simulink model "sampleModel1606_4_sub_sub"  (R2023a)
settings: Solver=VariableStepAuto  StartTime=0.0  StopTime=10.0  RelTol=1e-3
libraries: hdlsllib x6, simulink x3
settings Model: Creator=user1  LastModifiedBy=user1

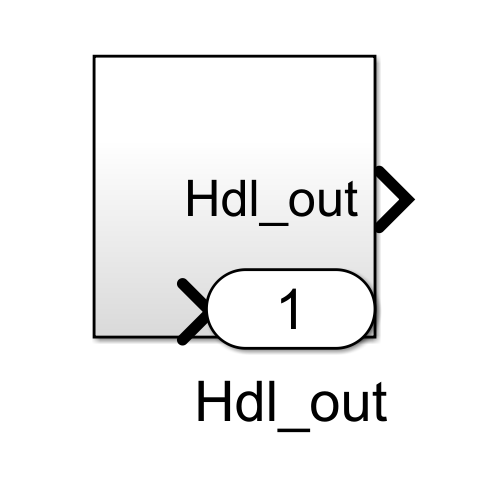
[thumbnail: Simulink's stored preview of the top-level diagram]
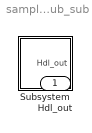
== system sampleModel1606_4_sub_sub ==
  Subsystem : Subsystem
  Hdl_out : Outport  OutDataTypeStr=uint8

== system sampleModel1606_4_sub_sub/Subsystem ==
  Subsystem : Subsystem
  Hdl_out : Outport  OutDataTypeStr=uint8

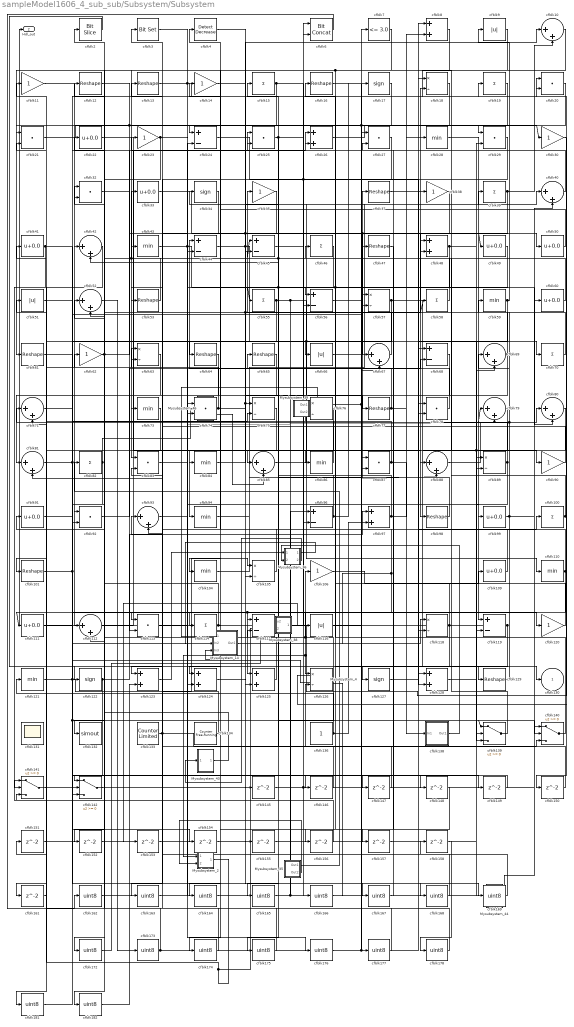
== system sampleModel1606_4_sub_sub/Subsystem/Subsystem ==
  Mysubsystem_14 : Subsystem  TreatAsAtomicUnit=on  RTWFcnName=Mysubsystem_14
      settings: RTWFcnNameOpts=User specified  RTWFileNameOpts=Use function name
  Mysubsystem_2 : Subsystem  TreatAsAtomicUnit=on  RTWFcnName=Mysubsystem_2
      settings: RTWFcnNameOpts=User specified  RTWFileNameOpts=Use function name
  Mysubsystem_35 : Subsystem  TreatAsAtomicUnit=on  RTWFcnName=Mysubsystem_35
      settings: RTWFcnNameOpts=User specified  RTWFileNameOpts=Use function name
  Mysubsystem_36 : Subsystem  TreatAsAtomicUnit=on  RTWFcnName=Mysubsystem_36
      settings: RTWFcnNameOpts=User specified  RTWFileNameOpts=Use function name
  Mysubsystem_38 : Subsystem  TreatAsAtomicUnit=on  RTWFcnName=Mysubsystem_38
      settings: RTWFcnNameOpts=User specified  RTWFileNameOpts=Use function name
  Mysubsystem_39 : Subsystem  TreatAsAtomicUnit=on  RTWFcnName=Mysubsystem_39
      settings: RTWFcnNameOpts=User specified  RTWFileNameOpts=Use function name
  Mysubsystem_4 : Subsystem  TreatAsAtomicUnit=on  RTWFcnName=Mysubsystem_4
      settings: RTWFcnNameOpts=User specified  RTWFileNameOpts=Use function name
  Mysubsystem_43 : Subsystem  TreatAsAtomicUnit=on  RTWFcnName=Mysubsystem_43
      settings: RTWFcnNameOpts=User specified  RTWFileNameOpts=Use function name
  Mysubsystem_44 : Subsystem  TreatAsAtomicUnit=on  RTWFcnName=Mysubsystem_44
      settings: RTWFcnNameOpts=User specified  RTWFileNameOpts=Use function name
  Mysubsystem_46 : Subsystem  TreatAsAtomicUnit=on  RTWFcnName=Mysubsystem_46
      settings: RTWFcnNameOpts=User specified  RTWFileNameOpts=Use function name
  cfblk{10,40,42,52,67,69,71,79..81,85,88,93,112} (14 alike) : Sum  Inputs=|++  OutDataTypeStr=uint8
  cfblk{15,19,39,46,55,58,70,82,100,114} (10 alike) : Sum  Inputs=+  OutDataTypeStr=uint8
  cfblk{12..13,16,37,47,53,61,64..65,77,98,101,129} (13 alike) : Reshape
  cfblk{28,43,59,73,84,86,94,104,110,121} (10 alike) : MinMax  OutDataTypeStr=uint8
  cfblk{18,57,63,75..76,89,105,118,126} (9 alike) : Product  Inputs=*/  OutDataTypeStr=uint8  RndMeth=Zero  SaturateOnIntegerOverflow=on
  cfblk{11,14,23,30,35,38,62,90,106,120} (10 alike) : Gain  OutDataTypeStr=uint8
  cfblk{22,33,41,49..50,60,91,99,109,111} (10 alike) : Bias  Bias=0.0  SaturateOnIntegerOverflow=off
  cfblk{20..21,25,27,29,32,74,78,83,87,92,113} (12 alike) : DotProduct  OutDataTypeStr=uint8
  cfblk{24,44..45,56,68,96,115,119} (8 alike) : Sum  Inputs=+-  OutDataTypeStr=uint8
  cfblk{9,51,66,116} (4 alike) : Abs  OutDataTypeStr=uint8  SaturateOnIntegerOverflow=off
  cfblk{17,34,122,127} (4 alike) : Signum
  cfblk{8,26,48,97,123..125,128} (8 alike) : Sum  OutDataTypeStr=uint8
  cfblk131 : Scope
      settings: Floating=on
  cfblk132 : ToWorkspace  VariableName=simout  SaveFormat=Timeseries  SampleTime=-1
  cfblk133 : hdlsllib/Sources/Counter Limited  uplimit=7  tsamp=-1
  cfblk134 : hdlsllib/Sources/Counter Free-Running  NumBits=16  tsamp=-1
  cfblk136 : Constant  OutDataTypeStr=uint8  SampleTime=-1
  cfblk138 : Subsystem
      settings: LibrarySourceBlock=|
      | hdlsllib/Ports &
      | Subsystems/Subsystem
  cfblk{139..142} (4 alike) : Switch  OutDataTypeStr=uint8  SaturateOnIntegerOverflow=off  InputSameDT=off
  cfblk{145..158,161} (15 alike) : Delay  SampleTime=1
  cfblk{162..169,172..178,181..182} (17 alike) : DataTypeConversion  OutDataTypeStr=uint8  SaturateOnIntegerOverflow=off  RndMeth=Floor
  cfblk2 : hdlsllib/Logic and Bit Operations/Bit Slice  lidx=7  ridx=0
  cfblk3 : simulink/Logic and Bit Operations/Bit Set  iBit=0
      settings: LibrarySourceBlock=|
      | hdlsllib/Logic and Bit
      | Operations/Bit Set
  cfblk4 : simulink/Logic and Bit Operations/Detect Decrease  vinit=0.0  OutDataTypeStr=uint8
      settings: LibrarySourceBlock=|
      | hdlsllib/Logic and Bit
      | Operations/Detect
      | Decrease
  cfblk6 : hdlsllib/Logic and Bit Operations/Bit Concat  numInputs=2
  cfblk7 : hdlsllib/Logic and Bit Operations/Compare To Constant  relop=<=  const=3.0  OutDataTypeStr=uint8
  cfblk130 : Outport  OutDataTypeStr=uint8  VectorParamsAs1DForOutWhenUnconnected=off
  Hdl_out : Outport  Port=2  OutDataTypeStr=uint8
  wires:
  Mysubsystem_46/1(Out1) -> cfblk85/2
  Mysubsystem_44/1(Out1) -> cfblk140/1
  Mysubsystem_4/1(Out1) -> Mysubsystem_44/1(In1)
  Mysubsystem_43/1(Out1) -> cfblk182/1
  Mysubsystem_36/2(Out2) -> Mysubsystem_43/1(In1)
  Mysubsystem_39/2(Out2) -> Mysubsystem_14/1(In1)
  Mysubsystem_39/1(Out1) -> cfblk19/1, cfblk88/2
  Mysubsystem_38/1(Out1) -> cfblk153/1
  cfblk172/1 -> Mysubsystem_38/1(u2)
  Mysubsystem_36/1(Out1) -> Mysubsystem_14/2(In2)
  cfblk138/1(Out1) -> Mysubsystem_36/2(In2)
  cfblk123/1 -> Mysubsystem_36/1(In1)
  Mysubsystem_35/2(Out2) -> Mysubsystem_2/2(In2)
  Mysubsystem_35/1(Out1) -> cfblk82/1
  Mysubsystem_14/1(Out1) -> cfblk81/2, Mysubsystem_2/1(In1), cfblk126/1
  cfblk181/1 -> Mysubsystem_4/2(In2)
  Mysubsystem_2/1(Out1) -> Mysubsystem_38/2(In2), cfblk141/3
  cfblk182/1 -> cfblk123/2
  cfblk73/1 -> cfblk181/1
  cfblk178/1 -> cfblk93/2
  cfblk158/1 -> cfblk178/1
  cfblk177/1 -> cfblk93/1
  cfblk16/1 -> cfblk177/1
  cfblk176/1 -> cfblk87/1, cfblk78/2
  cfblk175/1 -> cfblk52/2
  cfblk174/1 -> cfblk52/1
  cfblk35/1 -> cfblk174/1
  cfblk173/1 -> cfblk151/1, cfblk18/1
  cfblk169/1 -> cfblk158/1
  cfblk3/1 -> cfblk169/1
  cfblk168/1 -> cfblk3/1
  cfblk71/1 -> cfblk168/1
  cfblk167/1 -> cfblk27/2
  cfblk166/1 -> cfblk27/1
  cfblk165/1 -> cfblk69/2, cfblk96/1
  cfblk164/1 -> cfblk6/2
  cfblk148/1 -> cfblk164/1
  cfblk163/1 -> cfblk6/1
  cfblk68/1 -> cfblk163/1
  cfblk162/1 -> cfblk74/1
  cfblk6/1 -> cfblk162/1
  cfblk161/1 -> cfblk21/2
  cfblk157/1 -> cfblk128/1
  cfblk119/1 -> cfblk157/1, Hdl_out/1
  cfblk156/1 -> cfblk141/1
  cfblk155/1 -> cfblk78/1
  cfblk14/1 -> cfblk155/1
  cfblk154/1 -> cfblk89/1
  cfblk153/1 -> cfblk24/2
  cfblk152/1 -> cfblk68/1
  cfblk75/1 -> cfblk152/1
  cfblk151/1 -> cfblk74/2
  cfblk150/1 -> cfblk83/2
  cfblk30/1 -> cfblk150/1
  cfblk149/1 -> cfblk142/1
  cfblk61/1 -> cfblk149/1
  cfblk113/1 -> cfblk148/1
  cfblk147/1 -> cfblk115/2
  cfblk47/1 -> cfblk147/1
  cfblk146/1 -> cfblk126/2
  cfblk145/1 -> cfblk40/2
  cfblk124/1 -> cfblk145/1
  cfblk12/1 -> cfblk30/1, cfblk66/1
  cfblk64/1 -> cfblk92/1
  cfblk129/1 -> cfblk59/1, cfblk79/1
  cfblk116/1 -> cfblk57/1
  cfblk10/1 -> cfblk56/1, cfblk172/1
  cfblk34/1 -> cfblk53/1
  cfblk90/1 -> cfblk43/1
  cfblk141/1 -> cfblk118/1
  cfblk46/1 -> cfblk125/2
  cfblk139/1 -> cfblk48/1
  cfblk62/1 -> cfblk26/2, cfblk32/2
  cfblk53/1 -> cfblk12/1
  cfblk45/1 -> cfblk49/1, cfblk47/1
  cfblk82/1 -> Mysubsystem_46/1(In1), cfblk92/2
  cfblk133/1 -> cfblk63/2, cfblk140/3
  cfblk98/1 -> cfblk23/1
  cfblk128/1 -> cfblk140/2
  cfblk122/1 -> cfblk142/3, cfblk97/1
  cfblk69/1 -> cfblk32/1, cfblk71/2
  cfblk32/1 -> cfblk44/2
  cfblk109/1 -> cfblk63/1
  cfblk51/1 -> cfblk70/1
  cfblk4/1 -> cfblk75/1, cfblk167/1
  cfblk20/1 -> cfblk64/1
  cfblk101/1 -> cfblk130/1, cfblk75/2
  cfblk134/1 -> cfblk13/1
  cfblk83/1 -> cfblk96/2
  cfblk25/1 -> cfblk115/1, cfblk55/1, cfblk99/1
  cfblk74/1 -> cfblk51/1, cfblk77/1
  cfblk19/1 -> cfblk113/2, cfblk87/2
  cfblk48/1 -> cfblk124/2, cfblk50/1
  cfblk43/1 -> cfblk80/2, cfblk127/1
  cfblk96/1 -> cfblk34/1, cfblk45/1, cfblk17/1
  cfblk41/1 -> cfblk142/2, cfblk141/2
  cfblk97/1 -> cfblk42/2, cfblk28/1
  cfblk60/1 -> cfblk33/1, cfblk2/1
  cfblk50/1 -> cfblk14/1
  cfblk44/1 -> cfblk89/2, cfblk10/1
  cfblk110/1 -> cfblk125/1, cfblk111/1, cfblk71/1
  cfblk79/1 -> cfblk119/2, cfblk132/1
  cfblk66/1 -> cfblk67/2
  cfblk142/1 -> cfblk29/2, cfblk56/2
  cfblk106/1 -> cfblk109/1
  cfblk93/1 -> cfblk176/1
  cfblk49/1 -> cfblk124/1, cfblk146/1
  cfblk87/1 -> cfblk62/1, cfblk138/1(In1)
  cfblk29/1 -> cfblk113/1
  cfblk17/1 -> cfblk84/1
  cfblk15/1 -> cfblk21/1, cfblk88/1
  cfblk26/1 -> cfblk29/1
  cfblk33/1 -> cfblk67/1
  cfblk42/1 -> cfblk101/1
  cfblk111/1 -> cfblk20/2
  cfblk11/1 -> cfblk42/1
  cfblk40/1 -> cfblk25/1
  cfblk70/1 -> cfblk38/1
  cfblk92/1 -> cfblk68/2
  cfblk99/1 -> cfblk60/1, cfblk69/1
  cfblk114/1 -> Mysubsystem_14/3(In3), cfblk22/1
  cfblk125/1 -> cfblk91/1
  cfblk8/1 -> cfblk83/1
  cfblk38/1 -> cfblk123/1, cfblk45/2
  cfblk59/1 -> cfblk9/1, cfblk118/2
  cfblk127/1 -> cfblk100/1
  cfblk86/1 -> cfblk11/1
  cfblk84/1 -> cfblk39/1, cfblk58/1
  cfblk118/1 -> cfblk76/2, cfblk156/1
  cfblk22/1 -> cfblk85/1
  cfblk9/1 -> cfblk104/1
  cfblk65/1 -> cfblk114/1
  cfblk58/1 -> cfblk46/1
  cfblk81/1 -> cfblk120/1, cfblk57/2
  cfblk126/1 -> cfblk15/1, cfblk106/1, cfblk175/1
  cfblk120/1 -> cfblk76/1
  cfblk94/1 -> cfblk8/1
  cfblk21/1 -> cfblk24/1
  cfblk23/1 -> cfblk112/2, cfblk86/1
  cfblk77/1 -> cfblk44/1, cfblk8/2
  cfblk24/1 -> cfblk128/2, cfblk116/1
  cfblk140/1 -> cfblk16/1
  cfblk105/1 -> cfblk4/1
  cfblk91/1 -> cfblk139/1, cfblk154/1
  cfblk67/1 -> cfblk35/1
  cfblk115/1 -> cfblk20/1
  cfblk56/1 -> cfblk7/1
  cfblk39/1 -> cfblk98/1, cfblk10/2
  cfblk112/1 -> cfblk26/1
  cfblk85/1 -> cfblk40/1
  cfblk2/1 -> cfblk122/1
  cfblk89/1 -> cfblk41/1, cfblk139/3
  cfblk63/1 -> cfblk81/1
  cfblk57/1 -> cfblk90/1, cfblk161/1
  cfblk100/1 -> Mysubsystem_4/1(In1), cfblk48/2
  cfblk27/1 -> cfblk165/1
  cfblk136/1 -> cfblk121/1, cfblk97/2
  cfblk80/1 -> cfblk105/2
  cfblk78/1 -> cfblk65/1
  cfblk28/1 -> cfblk119/1
  cfblk55/1 -> cfblk110/1, cfblk139/2, cfblk166/1, cfblk73/1
  cfblk37/1 -> cfblk18/2
  cfblk52/1 -> cfblk173/1
  cfblk121/1 -> cfblk105/1, cfblk25/2
  cfblk104/1 -> cfblk37/1
  cfblk13/1 -> cfblk129/1, cfblk79/2
  cfblk88/1 -> cfblk80/1
  cfblk76/1 -> cfblk94/1
  cfblk7/1 -> cfblk61/1
  cfblk18/1 -> cfblk112/1

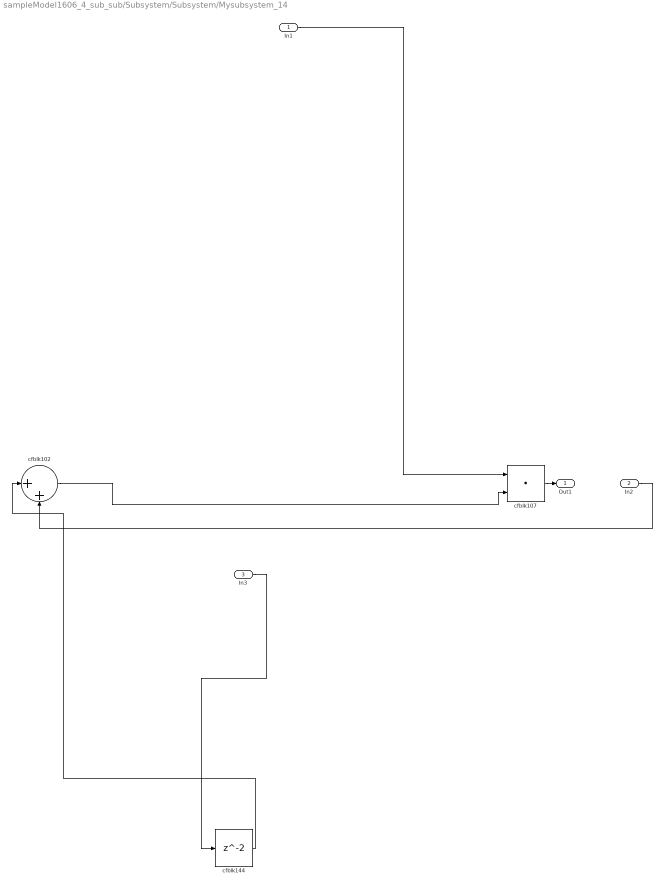
== system sampleModel1606_4_sub_sub/Subsystem/Subsystem/Mysubsystem_14 ==
  In1 : Inport
  In2 : Inport  Port=2
  In3 : Inport  Port=3
  cfblk102 : Sum  Inputs=|++
  cfblk107 : DotProduct  OutDataTypeStr=Inherit: Inherit via internal rule
  cfblk144 : Delay  SampleTime=1
  Out1 : Outport
  wires:
  cfblk102/1 -> cfblk107/2
  In2/1 -> cfblk102/2
  cfblk144/1 -> cfblk102/1
  In1/1 -> cfblk107/1
  cfblk107/1 -> Out1/1
  In3/1 -> cfblk144/1

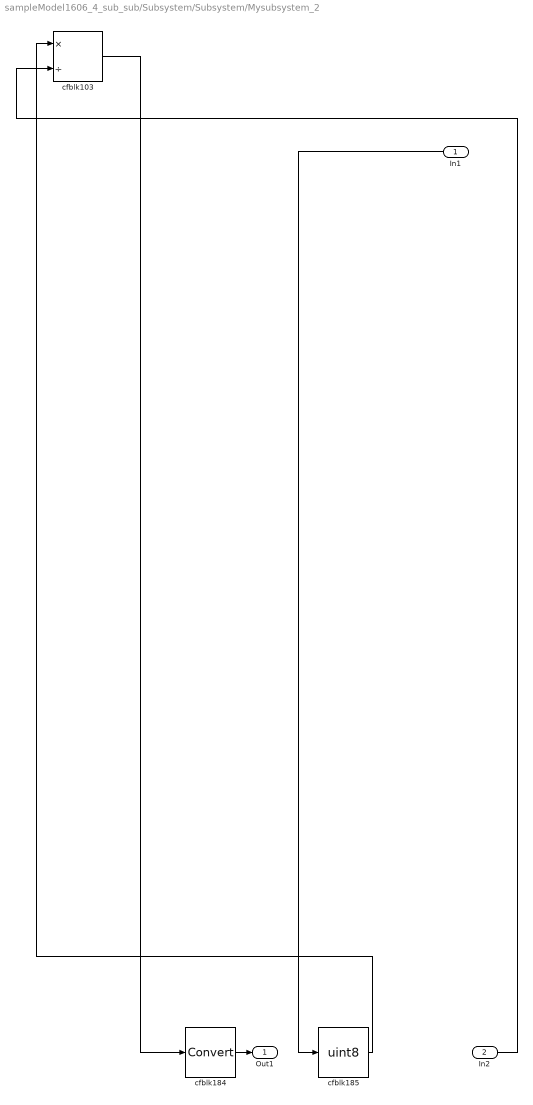
== system sampleModel1606_4_sub_sub/Subsystem/Subsystem/Mysubsystem_2 ==
  In1 : Inport
  In2 : Inport  Port=2
  cfblk103 : Product  Inputs=*/  RndMeth=Zero  SaturateOnIntegerOverflow=on
  cfblk184 : DataTypeConversion  SaturateOnIntegerOverflow=off  RndMeth=Floor
  cfblk185 : DataTypeConversion  OutDataTypeStr=uint8  SaturateOnIntegerOverflow=off  RndMeth=Floor
  Out1 : Outport
  wires:
  cfblk103/1 -> cfblk184/1
  cfblk185/1 -> cfblk103/1
  In2/1 -> cfblk103/2
  cfblk184/1 -> Out1/1
  In1/1 -> cfblk185/1

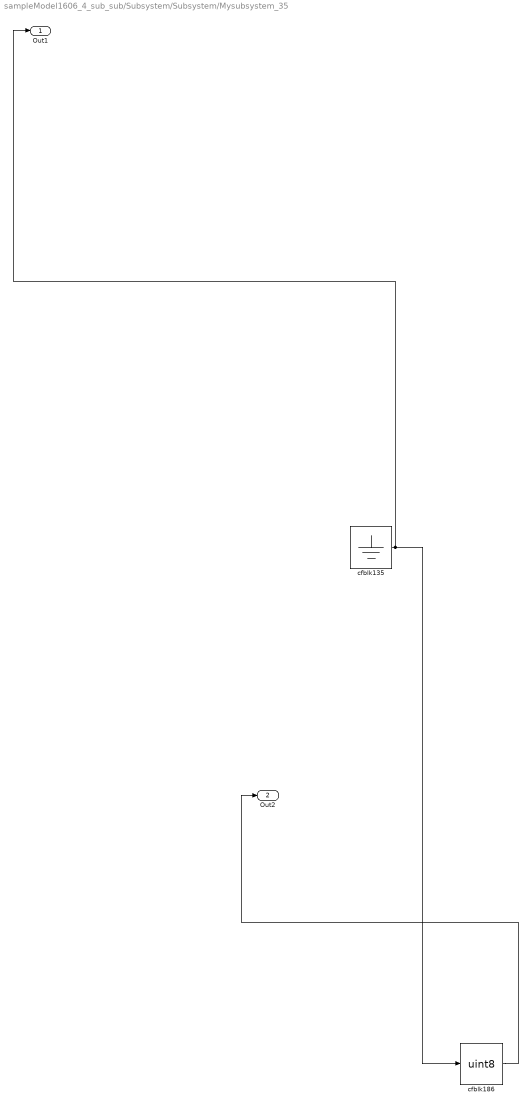
== system sampleModel1606_4_sub_sub/Subsystem/Subsystem/Mysubsystem_35 ==
  cfblk135 : Ground
  cfblk186 : DataTypeConversion  OutDataTypeStr=uint8  SaturateOnIntegerOverflow=off  RndMeth=Floor
  Out1 : Outport
  Out2 : Outport  Port=2
  wires:
  cfblk135/1 -> Out1/1, cfblk186/1
  cfblk186/1 -> Out2/1

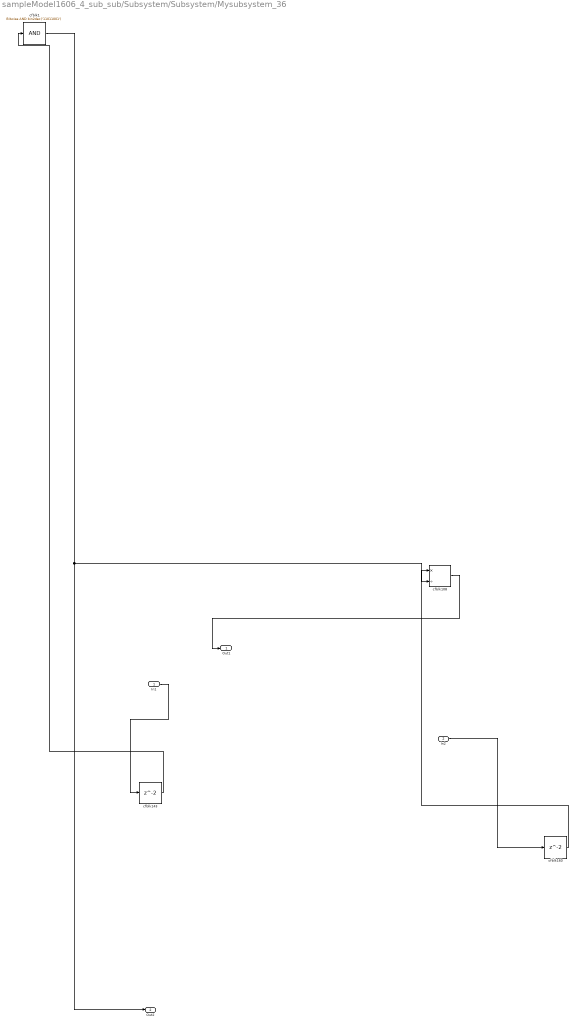
== system sampleModel1606_4_sub_sub/Subsystem/Subsystem/Mysubsystem_36 ==
  In1 : Inport
  In2 : Inport  Port=2
  cfblk1 : simulink/Logic and Bit Operations/Bitwise Operator  logicop=AND  UseBitMask=on  BitMask=bin2dec('11011001')  BitMaskRealWorld=Stored Integer
      settings: LibrarySourceBlock=|
      | hdlsllib/Logic and Bit
      | Operations/Bitwise
      | Operator
  cfblk108 : Product  Inputs=*/  RndMeth=Zero  SaturateOnIntegerOverflow=on
  cfblk143 : Delay  SampleTime=1
  cfblk160 : Delay  SampleTime=1
  Out1 : Outport
  Out2 : Outport  Port=2
  wires:
  cfblk1/1 -> Out2/1, cfblk108/2
  cfblk143/1 -> cfblk1/1
  cfblk160/1 -> cfblk108/1
  cfblk108/1 -> Out1/1
  In2/1 -> cfblk160/1
  In1/1 -> cfblk143/1

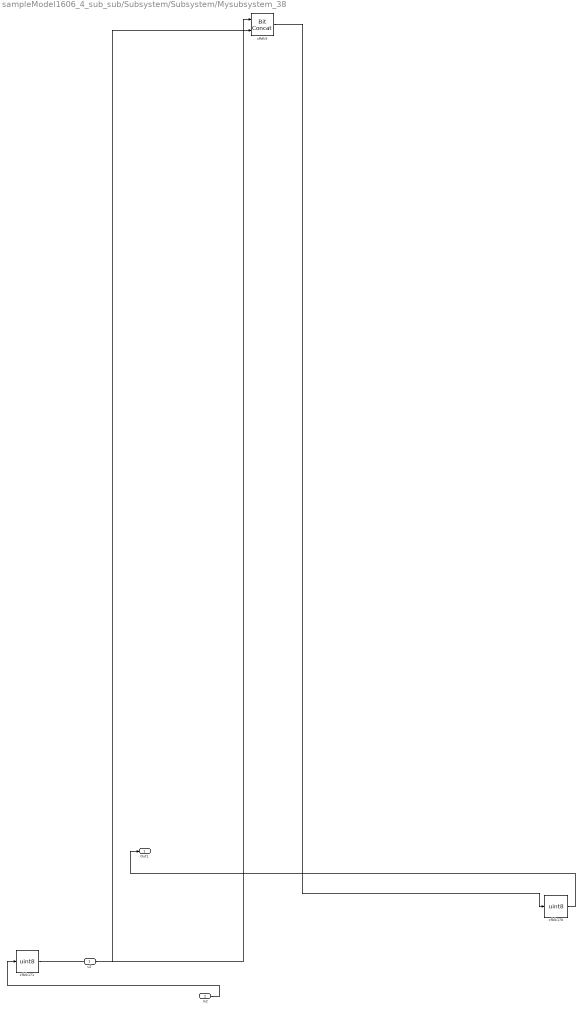
== system sampleModel1606_4_sub_sub/Subsystem/Subsystem/Mysubsystem_38 ==
  u2 : Inport
  In2 : Inport  Port=2
  cfblk170 : DataTypeConversion  OutDataTypeStr=uint8  SaturateOnIntegerOverflow=off  RndMeth=Floor
  cfblk171 : DataTypeConversion  OutDataTypeStr=uint8  SaturateOnIntegerOverflow=off  RndMeth=Floor
  cfblk5 : hdlsllib/Logic and Bit Operations/Bit Concat  numInputs=2
  Out1 : Outport
  wires:
  cfblk5/1 -> cfblk170/1
  cfblk171/1 -> cfblk5/1
  In2/1 -> cfblk171/1
  cfblk170/1 -> Out1/1
  u2/1 -> cfblk5/2

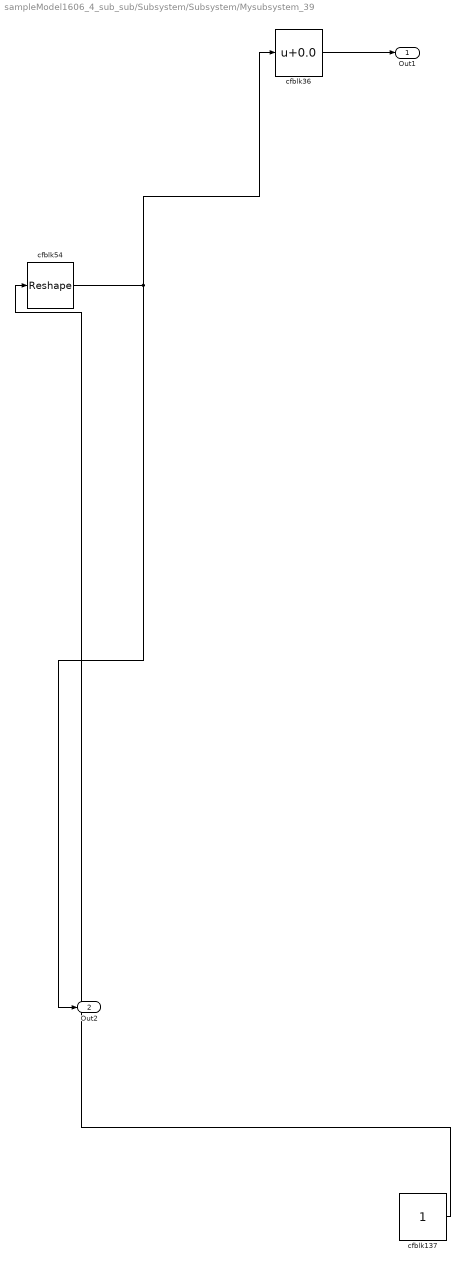
== system sampleModel1606_4_sub_sub/Subsystem/Subsystem/Mysubsystem_39 ==
  cfblk137 : Constant  SampleTime=-1
  cfblk36 : Bias  Bias=0.0  SaturateOnIntegerOverflow=off
  cfblk54 : Reshape
  Out1 : Outport
  Out2 : Outport  Port=2
  wires:
  cfblk36/1 -> Out1/1
  cfblk54/1 -> Out2/1, cfblk36/1
  cfblk137/1 -> cfblk54/1

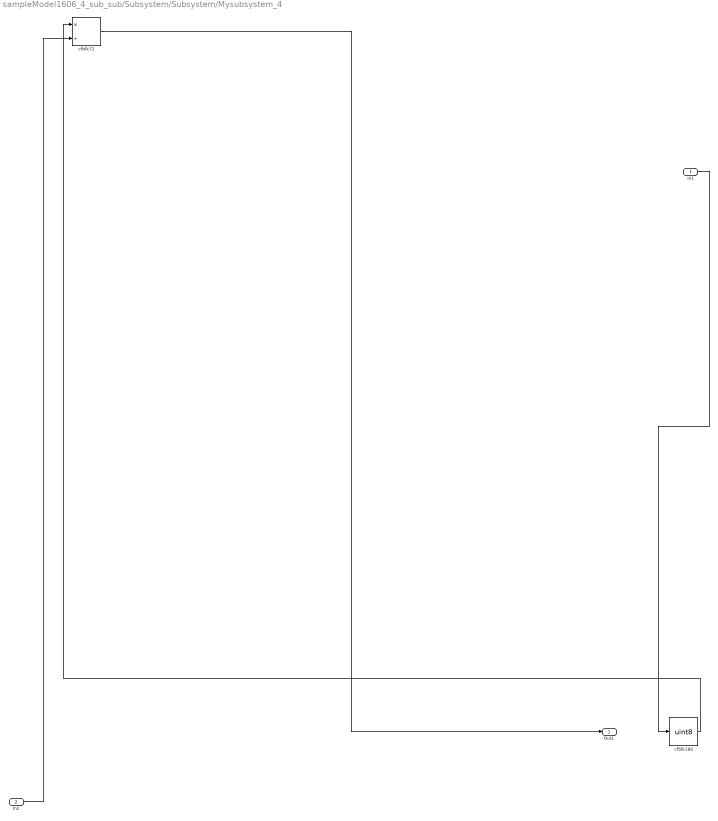
== system sampleModel1606_4_sub_sub/Subsystem/Subsystem/Mysubsystem_4 ==
  In1 : Inport
  In2 : Inport  Port=2
  cfblk180 : DataTypeConversion  OutDataTypeStr=uint8  SaturateOnIntegerOverflow=off  RndMeth=Floor
  cfblk72 : Product  Inputs=*/  RndMeth=Zero  SaturateOnIntegerOverflow=on
  Out1 : Outport
  wires:
  cfblk180/1 -> cfblk72/1
  In2/1 -> cfblk72/2
  In1/1 -> cfblk180/1
  cfblk72/1 -> Out1/1

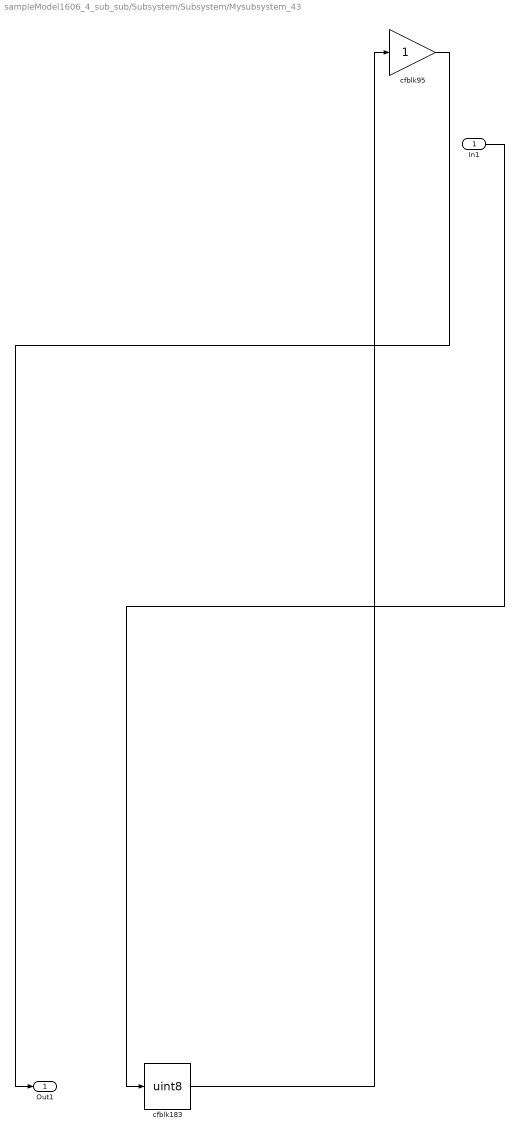
== system sampleModel1606_4_sub_sub/Subsystem/Subsystem/Mysubsystem_43 ==
  In1 : Inport
  cfblk183 : DataTypeConversion  OutDataTypeStr=uint8  SaturateOnIntegerOverflow=off  RndMeth=Floor
  cfblk95 : Gain
  Out1 : Outport
  wires:
  cfblk183/1 -> cfblk95/1
  In1/1 -> cfblk183/1
  cfblk95/1 -> Out1/1

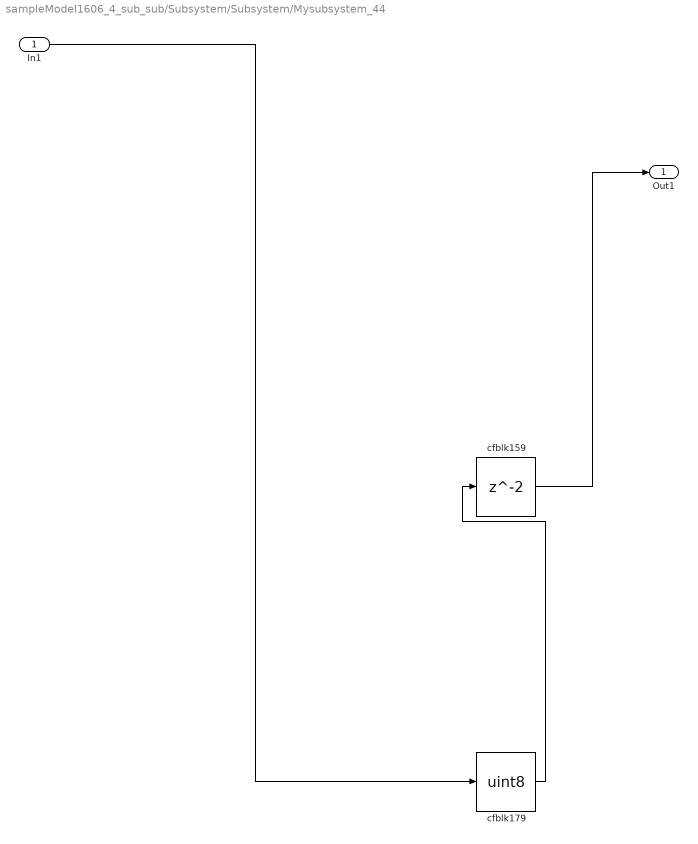
== system sampleModel1606_4_sub_sub/Subsystem/Subsystem/Mysubsystem_44 ==
  In1 : Inport
  cfblk159 : Delay  SampleTime=1
  cfblk179 : DataTypeConversion  OutDataTypeStr=uint8  SaturateOnIntegerOverflow=off  RndMeth=Floor
  Out1 : Outport
  wires:
  cfblk179/1 -> cfblk159/1
  In1/1 -> cfblk179/1
  cfblk159/1 -> Out1/1

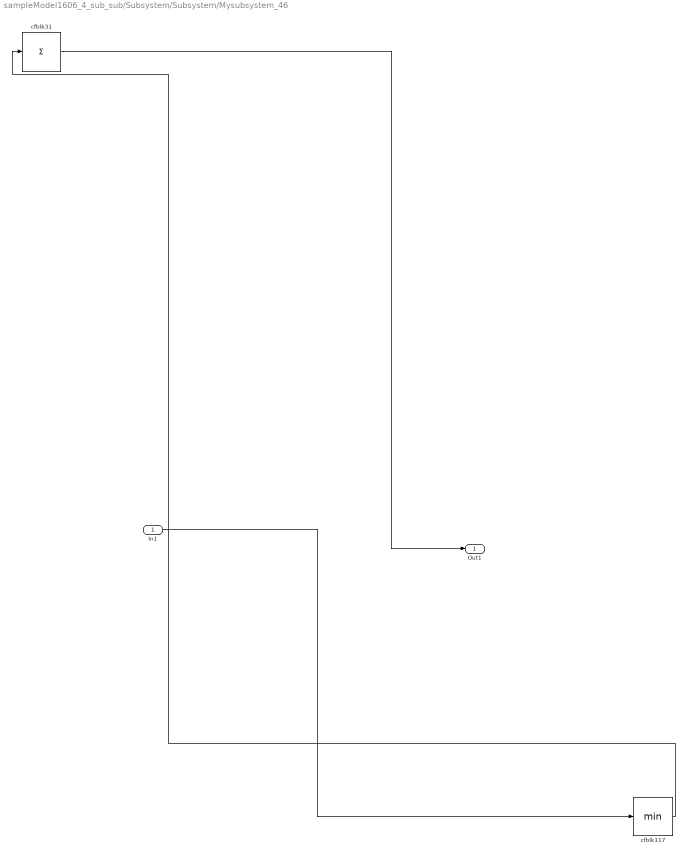
== system sampleModel1606_4_sub_sub/Subsystem/Subsystem/Mysubsystem_46 ==
  In1 : Inport
  cfblk117 : MinMax
  cfblk31 : Sum  Inputs=+
  Out1 : Outport
  wires:
  cfblk117/1 -> cfblk31/1
  cfblk31/1 -> Out1/1
  In1/1 -> cfblk117/1

== system sampleModel1606_4_sub_sub/Subsystem/Subsystem/cfblk138 ==
  In1 : Inport
  Out1 : Outport
  wires:
  In1/1 -> Out1/1
